simulink model "Ghost"  (Simulink 8.1)
settings: Solver=ode1  StartTime=0.0  StopTime=inf  FixedStep=Ts  MaxStep=1e-3  RelTol=1e-3
PostLoadFcn:
  | NREL_Mode=1; Ghost_init;
InitFcn:
  | NREL_Mode=1; Ghost_init;
undefined symbols (not defined in the file): Stim, Ts
libraries: simulink x75, artemis x11, relay_housing_lib x4, rtlab x1, utility_service_lib x1, communications_lib x1, Feeder1_lib x1, Feeder2_lib x1, Feeder3_lib x1, Feeder4_lib x1, powerlib x1
(part 2 of 2)

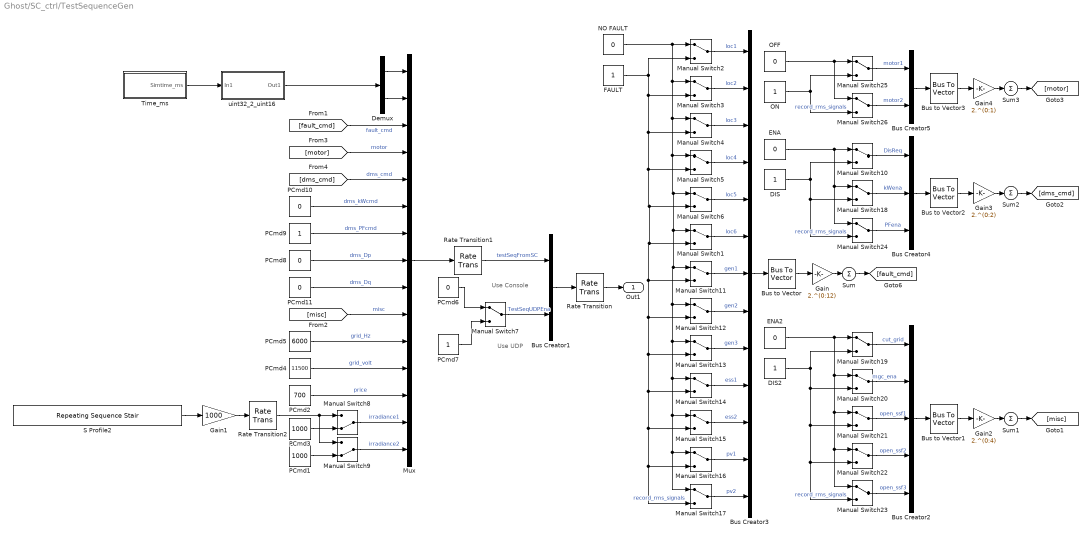
== system Ghost/SC_ctrl/TestSequenceGen ==
  note: Use UDP
  note: Use Console
  Bus Creator1 : BusCreator  Inputs=2
  Bus Creator2 : BusCreator  Inputs=5
  Bus Creator3 : BusCreator  Inputs=13
  Bus Creator4 : BusCreator  Inputs=3
  Bus Creator5 : BusCreator  Inputs=2
  Bus to Vector{,1..3} (4 alike) : BusToVector
  DIS : Constant
  DIS2 : Constant
  Demux : Demux  Outputs=2
  ENA : Constant  Value=0
  ENA2 : Constant  Value=0
  FAULT : Constant
  Gain : Gain  Gain=2.^(0:12)
  Gain1 : Gain  Gain=1000
  Gain2 : Gain  Gain=2.^(0:4)
  Gain3 : Gain  Gain=2.^(0:2)
  Gain4 : Gain  Gain=2.^(0:1)
  Manual Switch{1..7,10..26} (24 alike) : ManualSwitch
  Manual Switch8 : ManualSwitch  CurrentSetting=0
  Manual Switch9 : ManualSwitch  CurrentSetting=0
  Mux : Mux  Inputs=15
  NO FAULT : Constant  Value=0
  OFF : Constant  Value=0
  ON : Constant
  PCmd1 : Constant  Value=1000
  PCmd10 : Constant  Value=0
  PCmd11 : Constant  Value=0
  PCmd2 : Constant  Value=700
  PCmd3 : Constant  Value=1000
  PCmd4 : Constant  Value=11500
  PCmd5 : Constant  Value=6000
  PCmd6 : Constant  Value=0  SampleTime=[Stim.Ts Ts]
  PCmd7 : Constant
  PCmd8 : Constant  Value=0
  PCmd9 : Constant
  Rate Transition : RateTransition  Deterministic=off
  Rate Transition1 : RateTransition  Deterministic=off  OutPortSampleTime=10e-3
  Rate Transition2 : RateTransition  Deterministic=off  OutPortSampleTime=10e-3
  S Profile2 : simulink/Sources/Repeating Sequence Stair  OutValues=Stim.PV2.Irradiance  tsamp=[Stim.Ts Ts]  OutMin=[]  OutMax=[]  OutDataTypeStr=Inherit: Inherit via back propagation  OutDataType=fixdt(0,8)  ConRadixGroup=Best Precision: Vector-wise  OutScaling=2^-12
  Sum{,1..3} (4 alike) : Sum  Inputs=+
  Time_ms : Subsystem
  uint32_2_uint16 : Subsystem
      mask Display: disp('uint32_2_uint16');
  Out1 : Outport
  wires:
  Rate Transition1/1 -> Bus Creator1/1  "testSeqFromSC"
  uint32_2_uint16/1(Out1) -> Demux/1
  S Profile2/1 -> Gain1/1
  Sum3/1 -> [motor]
  Gain4/1 -> Sum3/1
  Bus to Vector3/1 -> Gain4/1
  OFF/1 -> Manual Switch26/1, Manual Switch25/1
  ON/1 -> Manual Switch25/2, Manual Switch26/2  "record_rms_signals"
  Manual Switch26/1 -> Bus Creator5/2  "motor2"
  Manual Switch25/1 -> Bus Creator5/1  "motor1"
  Bus Creator5/1 -> Bus to Vector3/1
  Sum2/1 -> [dms_cmd]
  Gain3/1 -> Sum2/1
  Bus to Vector2/1 -> Gain3/1
  ENA/1 -> Manual Switch10/1, Manual Switch18/1, Manual Switch24/1
  DIS/1 -> Manual Switch18/2, Manual Switch24/2, Manual Switch10/2  "record_rms_signals"
  Manual Switch18/1 -> Bus Creator4/2  "kWena"
  Manual Switch10/1 -> Bus Creator4/1  "DisReq"
  Bus Creator4/1 -> Bus to Vector2/1
  Manual Switch24/1 -> Bus Creator4/3  "PFena"
  Sum1/1 -> [misc]
  Gain2/1 -> Sum1/1
  Bus to Vector1/1 -> Gain2/1
  ENA2/1 -> Manual Switch23/1, Manual Switch22/1, Manual Switch21/1, Manual Switch20/1, Manual Switch19/1
  DIS2/1 -> Manual Switch19/2, Manual Switch23/2, Manual Switch22/2, Manual Switch21/2, Manual Switch20/2  "record_rms_signals"
  Manual Switch20/1 -> Bus Creator2/2  "mgc_ena"
  Manual Switch23/1 -> Bus Creator2/5  "open_ssf3"
  Manual Switch19/1 -> Bus Creator2/1  "cut_grid"
  Bus Creator2/1 -> Bus to Vector1/1
  Manual Switch22/1 -> Bus Creator2/4  "open_ssf2"
  Manual Switch21/1 -> Bus Creator2/3  "open_ssf1"
  PCmd11/1 -> Mux/9  "dms_Dq"
  PCmd10/1 -> Mux/6  "dms_kWcmd"
  PCmd9/1 -> Mux/7  "dms_PFcmd"
  PCmd8/1 -> Mux/8  "dms_Dp"
  [dms_cmd] -> Mux/5  "dms_cmd"
  [motor] -> Mux/4  "motor"
  [misc] -> Mux/10  "misc"
  PCmd5/1 -> Mux/11  "grid_Hz"
  PCmd4/1 -> Mux/12  "grid_volt"
  Demux/2 -> Mux/2
  Demux/1 -> Mux/1
  Time_ms/1(Simtime_ms) -> uint32_2_uint16/1(In1)
  Gain1/1 -> Rate Transition2/1
  PCmd2/1 -> Mux/13  "price"
  Manual Switch8/1 -> Mux/14  "irradiance1"
  PCmd1/1 -> Manual Switch9/2
  Manual Switch9/1 -> Mux/15  "irradiance2"
  PCmd3/1 -> Manual Switch8/2
  Rate Transition/1 -> Out1/1
  PCmd7/1 -> Manual Switch7/2
  PCmd6/1 -> Manual Switch7/1
  Manual Switch7/1 -> Bus Creator1/2  "TestSeqUDPEna"
  Bus Creator1/1 -> Rate Transition/1
  Mux/1 -> Rate Transition1/1
  Sum/1 -> [fault_cmd]
  Gain/1 -> Sum/1
  Bus to Vector/1 -> Gain/1
  Manual Switch17/1 -> Bus Creator3/13  "pv2"
  Manual Switch16/1 -> Bus Creator3/12  "pv1"
  NO FAULT/1 -> Manual Switch2/1, Manual Switch3/1, Manual Switch4/1, Manual Switch5/1, Manual Switch6/1, Manual Switch1/1, Manual Switch11/1, Manual Switch16/1, Manual Switch17/1, Manual Switch15/1, Manual Switch14/1, Manual Switch13/1, Manual Switch12/1
  FAULT/1 -> Manual Switch3/2, Manual Switch4/2, Manual Switch5/2, Manual Switch6/2, Manual Switch11/2, Manual Switch15/2, Manual Switch16/2, Manual Switch17/2, Manual Switch14/2, Manual Switch13/2, Manual Switch12/2, Manual Switch1/2, Manual Switch2/2  "record_rms_signals"
  Manual Switch12/1 -> Bus Creator3/8  "gen2"
  Manual Switch15/1 -> Bus Creator3/11  "ess2"
  Manual Switch11/1 -> Bus Creator3/7  "gen1"
  Manual Switch14/1 -> Bus Creator3/10  "ess1"
  Manual Switch13/1 -> Bus Creator3/9  "gen3"
  Manual Switch1/1 -> Bus Creator3/6  "loc6"
  Manual Switch3/1 -> Bus Creator3/2  "loc2"
  Manual Switch6/1 -> Bus Creator3/5  "loc5"
  Manual Switch2/1 -> Bus Creator3/1  "loc1"
  Bus Creator3/1 -> Bus to Vector/1
  [fault_cmd] -> Mux/3  "fault_cmd"
  Manual Switch5/1 -> Bus Creator3/4  "loc4"
  Manual Switch4/1 -> Bus Creator3/3  "loc3"
  Rate Transition2/1 -> Manual Switch8/1, Manual Switch9/1

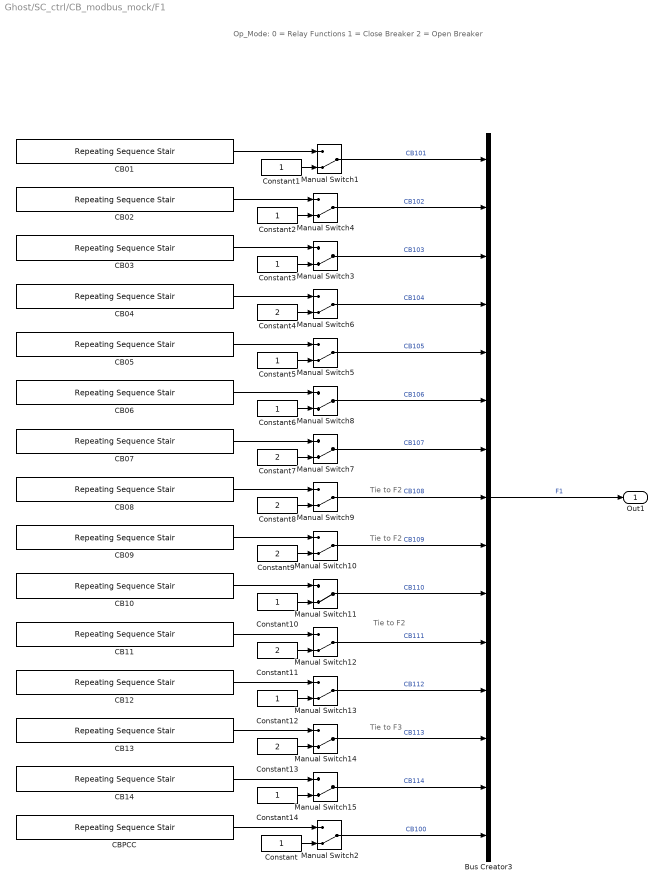
== system Ghost/SC_ctrl/CB_modbus_mock/F1 ==
  note: Tie to F2
  note: Tie to F2
  note: Op_Mode:
      | 0 = Relay Functions
      | 1 = Close Breaker
      | 2 = Open Breaker
  note: Tie to F2
  note: Tie to F3
  Bus Creator3 : BusCreator  Inputs=15
  CB01 : simulink/Sources/Repeating Sequence Stair  OutValues=Stim.CB.CB101  tsamp=[Stim.Ts Ts]  OutMin=[]  OutMax=[]  OutDataTypeStr=Inherit: Inherit via back propagation  OutDataType=fixdt(0,8)  ConRadixGroup=Best Precision: Vector-wise  OutScaling=2^-12
  CB02 : simulink/Sources/Repeating Sequence Stair  OutValues=Stim.CB.CB102  tsamp=[Stim.Ts Ts]  OutMin=[]  OutMax=[]  OutDataTypeStr=Inherit: Inherit via back propagation  OutDataType=fixdt(0,8)  ConRadixGroup=Best Precision: Vector-wise  OutScaling=2^-12
  CB03 : simulink/Sources/Repeating Sequence Stair  OutValues=Stim.CB.CB103  tsamp=[Stim.Ts Ts]  OutMin=[]  OutMax=[]  OutDataTypeStr=Inherit: Inherit via back propagation  OutDataType=fixdt(0,8)  ConRadixGroup=Best Precision: Vector-wise  OutScaling=2^-12
  CB04 : simulink/Sources/Repeating Sequence Stair  OutValues=Stim.CB.CB104  tsamp=[Stim.Ts Ts]  OutMin=[]  OutMax=[]  OutDataTypeStr=Inherit: Inherit via back propagation  OutDataType=fixdt(0,8)  ConRadixGroup=Best Precision: Vector-wise  OutScaling=2^-12
  CB05 : simulink/Sources/Repeating Sequence Stair  OutValues=Stim.CB.CB105  tsamp=[Stim.Ts Ts]  OutMin=[]  OutMax=[]  OutDataTypeStr=Inherit: Inherit via back propagation  OutDataType=fixdt(0,8)  ConRadixGroup=Best Precision: Vector-wise  OutScaling=2^-12
  CB06 : simulink/Sources/Repeating Sequence Stair  OutValues=Stim.CB.CB106  tsamp=[Stim.Ts Ts]  OutMin=[]  OutMax=[]  OutDataTypeStr=Inherit: Inherit via back propagation  OutDataType=fixdt(0,8)  ConRadixGroup=Best Precision: Vector-wise  OutScaling=2^-12
  CB07 : simulink/Sources/Repeating Sequence Stair  OutValues=Stim.CB.CB107  tsamp=[Stim.Ts Ts]  OutMin=[]  OutMax=[]  OutDataTypeStr=Inherit: Inherit via back propagation  OutDataType=fixdt(0,8)  ConRadixGroup=Best Precision: Vector-wise  OutScaling=2^-12
  CB08 : simulink/Sources/Repeating Sequence Stair  OutValues=Stim.CB.CB108  tsamp=[Stim.Ts Ts]  OutMin=[]  OutMax=[]  OutDataTypeStr=Inherit: Inherit via back propagation  OutDataType=fixdt(0,8)  ConRadixGroup=Best Precision: Vector-wise  OutScaling=2^-12
  CB09 : simulink/Sources/Repeating Sequence Stair  OutValues=Stim.CB.CB109  tsamp=[Stim.Ts Ts]  OutMin=[]  OutMax=[]  OutDataTypeStr=Inherit: Inherit via back propagation  OutDataType=fixdt(0,8)  ConRadixGroup=Best Precision: Vector-wise  OutScaling=2^-12
  CB10 : simulink/Sources/Repeating Sequence Stair  OutValues=Stim.CB.CB110  tsamp=[Stim.Ts Ts]  OutMin=[]  OutMax=[]  OutDataTypeStr=Inherit: Inherit via back propagation  OutDataType=fixdt(0,8)  ConRadixGroup=Best Precision: Vector-wise  OutScaling=2^-12
  CB11 : simulink/Sources/Repeating Sequence Stair  OutValues=Stim.CB.CB111  tsamp=[Stim.Ts Ts]  OutMin=[]  OutMax=[]  OutDataTypeStr=Inherit: Inherit via back propagation  OutDataType=fixdt(0,8)  ConRadixGroup=Best Precision: Vector-wise  OutScaling=2^-12
  CB12 : simulink/Sources/Repeating Sequence Stair  OutValues=Stim.CB.CB112  tsamp=[Stim.Ts Ts]  OutMin=[]  OutMax=[]  OutDataTypeStr=Inherit: Inherit via back propagation  OutDataType=fixdt(0,8)  ConRadixGroup=Best Precision: Vector-wise  OutScaling=2^-12
  CB13 : simulink/Sources/Repeating Sequence Stair  OutValues=Stim.CB.CB113  tsamp=[Stim.Ts Ts]  OutMin=[]  OutMax=[]  OutDataTypeStr=Inherit: Inherit via back propagation  OutDataType=fixdt(0,8)  ConRadixGroup=Best Precision: Vector-wise  OutScaling=2^-12
  CB14 : simulink/Sources/Repeating Sequence Stair  OutValues=Stim.CB.CB114  tsamp=[Stim.Ts Ts]  OutMin=[]  OutMax=[]  OutDataTypeStr=Inherit: Inherit via back propagation  OutDataType=fixdt(0,8)  ConRadixGroup=Best Precision: Vector-wise  OutScaling=2^-12
  CBPCC : simulink/Sources/Repeating Sequence Stair  OutValues=Stim.CB.CB100  tsamp=[Stim.Ts Ts]  OutMin=[]  OutMax=[]  OutDataTypeStr=Inherit: Inherit via back propagation  OutDataType=fixdt(0,8)  ConRadixGroup=Best Precision: Vector-wise  OutScaling=2^-12
  Constant{,1..3,5..6,10,12,14} (9 alike) : Constant
  Constant{4,7..9,11,13} (6 alike) : Constant  Value=2
  Manual Switch{1..15} (15 alike) : ManualSwitch  CurrentSetting=0
  Out1 : Outport
  wires:
  CB08/1 -> Manual Switch9/1
  Constant8/1 -> Manual Switch9/2
  Constant9/1 -> Manual Switch10/2
  Manual Switch9/1 -> Bus Creator3/8  "CB108"
  CB02/1 -> Manual Switch4/1
  Constant1/1 -> Manual Switch1/2
  Constant7/1 -> Manual Switch7/2
  Constant6/1 -> Manual Switch8/2
  CB07/1 -> Manual Switch7/1
  CB09/1 -> Manual Switch10/1
  Constant2/1 -> Manual Switch4/2
  CB06/1 -> Manual Switch8/1
  CB05/1 -> Manual Switch5/1
  Constant4/1 -> Manual Switch6/2
  Constant5/1 -> Manual Switch5/2
  CB04/1 -> Manual Switch6/1
  Manual Switch10/1 -> Bus Creator3/9  "CB109"
  Manual Switch8/1 -> Bus Creator3/6  "CB106"
  Manual Switch5/1 -> Bus Creator3/5  "CB105"
  Manual Switch6/1 -> Bus Creator3/4  "CB104"
  Manual Switch4/1 -> Bus Creator3/2  "CB102"
  Manual Switch1/1 -> Bus Creator3/1  "CB101"
  Manual Switch3/1 -> Bus Creator3/3  "CB103"
  Manual Switch7/1 -> Bus Creator3/7  "CB107"
  Manual Switch2/1 -> Bus Creator3/15  "CB100"
  Constant/1 -> Manual Switch2/2
  CBPCC/1 -> Manual Switch2/1
  CB01/1 -> Manual Switch1/1
  Bus Creator3/1 -> Out1/1  "F1"
  CB03/1 -> Manual Switch3/1
  Constant3/1 -> Manual Switch3/2
  Constant10/1 -> Manual Switch11/2
  CB10/1 -> Manual Switch11/1
  Manual Switch11/1 -> Bus Creator3/10  "CB110"
  Constant11/1 -> Manual Switch12/2
  CB11/1 -> Manual Switch12/1
  Manual Switch12/1 -> Bus Creator3/11  "CB111"
  Constant12/1 -> Manual Switch13/2
  CB12/1 -> Manual Switch13/1
  Manual Switch13/1 -> Bus Creator3/12  "CB112"
  Constant13/1 -> Manual Switch14/2
  CB13/1 -> Manual Switch14/1
  Manual Switch14/1 -> Bus Creator3/13  "CB113"
  Constant14/1 -> Manual Switch15/2
  CB14/1 -> Manual Switch15/1
  Manual Switch15/1 -> Bus Creator3/14  "CB114"

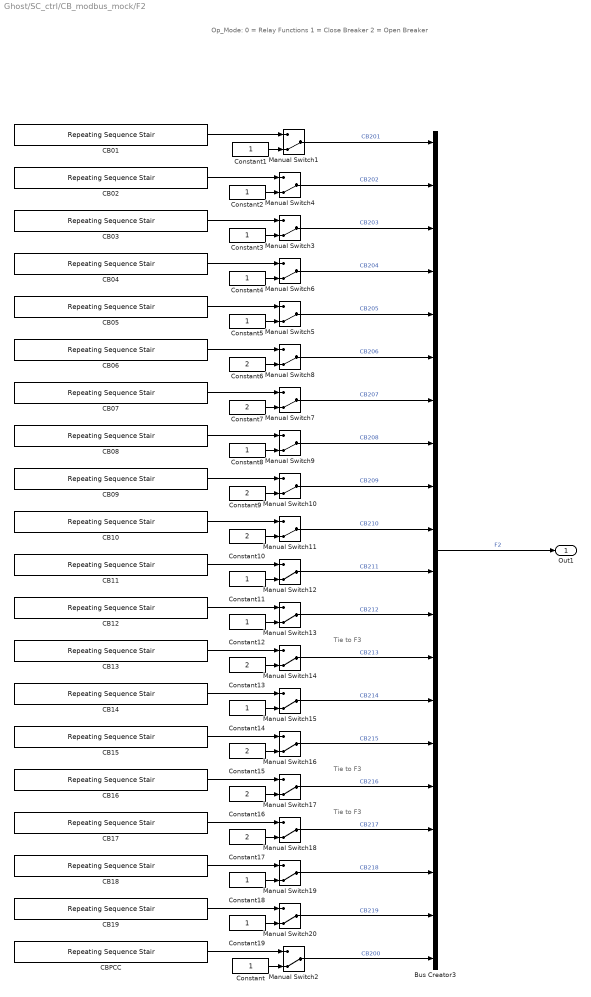
== system Ghost/SC_ctrl/CB_modbus_mock/F2 ==
  note: Tie to F3
  note: Op_Mode:
      | 0 = Relay Functions
      | 1 = Close Breaker
      | 2 = Open Breaker
  note: Tie to F3
  note: Tie to F3
  Bus Creator3 : BusCreator  Inputs=20
  CB01 : simulink/Sources/Repeating Sequence Stair  OutValues=Stim.CB.CB201  tsamp=[Stim.Ts Ts]  OutMin=[]  OutMax=[]  OutDataTypeStr=Inherit: Inherit via back propagation  OutDataType=fixdt(0,8)  ConRadixGroup=Best Precision: Vector-wise  OutScaling=2^-12
  CB02 : simulink/Sources/Repeating Sequence Stair  OutValues=Stim.CB.CB202  tsamp=[Stim.Ts Ts]  OutMin=[]  OutMax=[]  OutDataTypeStr=Inherit: Inherit via back propagation  OutDataType=fixdt(0,8)  ConRadixGroup=Best Precision: Vector-wise  OutScaling=2^-12
  CB03 : simulink/Sources/Repeating Sequence Stair  OutValues=Stim.CB.CB203  tsamp=[Stim.Ts Ts]  OutMin=[]  OutMax=[]  OutDataTypeStr=Inherit: Inherit via back propagation  OutDataType=fixdt(0,8)  ConRadixGroup=Best Precision: Vector-wise  OutScaling=2^-12
  CB04 : simulink/Sources/Repeating Sequence Stair  OutValues=Stim.CB.CB204  tsamp=[Stim.Ts Ts]  OutMin=[]  OutMax=[]  OutDataTypeStr=Inherit: Inherit via back propagation  OutDataType=fixdt(0,8)  ConRadixGroup=Best Precision: Vector-wise  OutScaling=2^-12
  CB05 : simulink/Sources/Repeating Sequence Stair  OutValues=Stim.CB.CB205  tsamp=[Stim.Ts Ts]  OutMin=[]  OutMax=[]  OutDataTypeStr=Inherit: Inherit via back propagation  OutDataType=fixdt(0,8)  ConRadixGroup=Best Precision: Vector-wise  OutScaling=2^-12
  CB06 : simulink/Sources/Repeating Sequence Stair  OutValues=Stim.CB.CB206  tsamp=[Stim.Ts Ts]  OutMin=[]  OutMax=[]  OutDataTypeStr=Inherit: Inherit via back propagation  OutDataType=fixdt(0,8)  ConRadixGroup=Best Precision: Vector-wise  OutScaling=2^-12
  CB07 : simulink/Sources/Repeating Sequence Stair  OutValues=Stim.CB.CB207  tsamp=[Stim.Ts Ts]  OutMin=[]  OutMax=[]  OutDataTypeStr=Inherit: Inherit via back propagation  OutDataType=fixdt(0,8)  ConRadixGroup=Best Precision: Vector-wise  OutScaling=2^-12
  CB08 : simulink/Sources/Repeating Sequence Stair  OutValues=Stim.CB.CB208  tsamp=[Stim.Ts Ts]  OutMin=[]  OutMax=[]  OutDataTypeStr=Inherit: Inherit via back propagation  OutDataType=fixdt(0,8)  ConRadixGroup=Best Precision: Vector-wise  OutScaling=2^-12
  CB09 : simulink/Sources/Repeating Sequence Stair  OutValues=Stim.CB.CB209  tsamp=[Stim.Ts Ts]  OutMin=[]  OutMax=[]  OutDataTypeStr=Inherit: Inherit via back propagation  OutDataType=fixdt(0,8)  ConRadixGroup=Best Precision: Vector-wise  OutScaling=2^-12
  CB10 : simulink/Sources/Repeating Sequence Stair  OutValues=Stim.CB.CB210  tsamp=[Stim.Ts Ts]  OutMin=[]  OutMax=[]  OutDataTypeStr=Inherit: Inherit via back propagation  OutDataType=fixdt(0,8)  ConRadixGroup=Best Precision: Vector-wise  OutScaling=2^-12
  CB11 : simulink/Sources/Repeating Sequence Stair  OutValues=Stim.CB.CB211  tsamp=[Stim.Ts Ts]  OutMin=[]  OutMax=[]  OutDataTypeStr=Inherit: Inherit via back propagation  OutDataType=fixdt(0,8)  ConRadixGroup=Best Precision: Vector-wise  OutScaling=2^-12
  CB12 : simulink/Sources/Repeating Sequence Stair  OutValues=Stim.CB.CB212  tsamp=[Stim.Ts Ts]  OutMin=[]  OutMax=[]  OutDataTypeStr=Inherit: Inherit via back propagation  OutDataType=fixdt(0,8)  ConRadixGroup=Best Precision: Vector-wise  OutScaling=2^-12
  CB13 : simulink/Sources/Repeating Sequence Stair  OutValues=Stim.CB.CB213  tsamp=[Stim.Ts Ts]  OutMin=[]  OutMax=[]  OutDataTypeStr=Inherit: Inherit via back propagation  OutDataType=fixdt(0,8)  ConRadixGroup=Best Precision: Vector-wise  OutScaling=2^-12
  CB14 : simulink/Sources/Repeating Sequence Stair  OutValues=Stim.CB.CB214  tsamp=[Stim.Ts Ts]  OutMin=[]  OutMax=[]  OutDataTypeStr=Inherit: Inherit via back propagation  OutDataType=fixdt(0,8)  ConRadixGroup=Best Precision: Vector-wise  OutScaling=2^-12
  CB15 : simulink/Sources/Repeating Sequence Stair  OutValues=Stim.CB.CB215  tsamp=[Stim.Ts Ts]  OutMin=[]  OutMax=[]  OutDataTypeStr=Inherit: Inherit via back propagation  OutDataType=fixdt(0,8)  ConRadixGroup=Best Precision: Vector-wise  OutScaling=2^-12
  CB16 : simulink/Sources/Repeating Sequence Stair  OutValues=Stim.CB.CB216  tsamp=[Stim.Ts Ts]  OutMin=[]  OutMax=[]  OutDataTypeStr=Inherit: Inherit via back propagation  OutDataType=fixdt(0,8)  ConRadixGroup=Best Precision: Vector-wise  OutScaling=2^-12
  CB17 : simulink/Sources/Repeating Sequence Stair  OutValues=Stim.CB.CB217  tsamp=[Stim.Ts Ts]  OutMin=[]  OutMax=[]  OutDataTypeStr=Inherit: Inherit via back propagation  OutDataType=fixdt(0,8)  ConRadixGroup=Best Precision: Vector-wise  OutScaling=2^-12
  CB18 : simulink/Sources/Repeating Sequence Stair  OutValues=Stim.CB.CB218  tsamp=[Stim.Ts Ts]  OutMin=[]  OutMax=[]  OutDataTypeStr=Inherit: Inherit via back propagation  OutDataType=fixdt(0,8)  ConRadixGroup=Best Precision: Vector-wise  OutScaling=2^-12
  CB19 : simulink/Sources/Repeating Sequence Stair  OutValues=Stim.CB.CB219  tsamp=[Stim.Ts Ts]  OutMin=[]  OutMax=[]  OutDataTypeStr=Inherit: Inherit via back propagation  OutDataType=fixdt(0,8)  ConRadixGroup=Best Precision: Vector-wise  OutScaling=2^-12
  CBPCC : simulink/Sources/Repeating Sequence Stair  OutValues=Stim.CB.CB200  tsamp=[Stim.Ts Ts]  OutMin=[]  OutMax=[]  OutDataTypeStr=Inherit: Inherit via back propagation  OutDataType=fixdt(0,8)  ConRadixGroup=Best Precision: Vector-wise  OutScaling=2^-12
  Constant{,1..5,8,11..12,14,18..19} (12 alike) : Constant
  Constant{6..7,9..10,13,15..17} (8 alike) : Constant  Value=2
  Manual Switch{1..20} (20 alike) : ManualSwitch  CurrentSetting=0
  Out1 : Outport
  wires:
  Manual Switch15/1 -> Bus Creator3/14  "CB214"
  CB14/1 -> Manual Switch15/1
  Constant14/1 -> Manual Switch15/2
  Manual Switch14/1 -> Bus Creator3/13  "CB213"
  CB13/1 -> Manual Switch14/1
  Constant13/1 -> Manual Switch14/2
  Manual Switch13/1 -> Bus Creator3/12  "CB212"
  CB12/1 -> Manual Switch13/1
  Constant12/1 -> Manual Switch13/2
  Manual Switch12/1 -> Bus Creator3/11  "CB211"
  CB11/1 -> Manual Switch12/1
  Constant11/1 -> Manual Switch12/2
  Manual Switch11/1 -> Bus Creator3/10  "CB210"
  CB10/1 -> Manual Switch11/1
  Constant10/1 -> Manual Switch11/2
  Constant3/1 -> Manual Switch3/2
  CB03/1 -> Manual Switch3/1
  Bus Creator3/1 -> Out1/1  "F2"
  CB01/1 -> Manual Switch1/1
  CBPCC/1 -> Manual Switch2/1
  Constant/1 -> Manual Switch2/2
  Manual Switch2/1 -> Bus Creator3/20  "CB200"
  Manual Switch7/1 -> Bus Creator3/7  "CB207"
  Manual Switch3/1 -> Bus Creator3/3  "CB203"
  Manual Switch1/1 -> Bus Creator3/1  "CB201"
  Manual Switch4/1 -> Bus Creator3/2  "CB202"
  Manual Switch6/1 -> Bus Creator3/4  "CB204"
  Manual Switch5/1 -> Bus Creator3/5  "CB205"
  Manual Switch8/1 -> Bus Creator3/6  "CB206"
  Manual Switch10/1 -> Bus Creator3/9  "CB209"
  CB04/1 -> Manual Switch6/1
  Constant5/1 -> Manual Switch5/2
  Constant4/1 -> Manual Switch6/2
  CB05/1 -> Manual Switch5/1
  CB06/1 -> Manual Switch8/1
  Constant2/1 -> Manual Switch4/2
  CB09/1 -> Manual Switch10/1
  CB07/1 -> Manual Switch7/1
  Constant6/1 -> Manual Switch8/2
  Constant7/1 -> Manual Switch7/2
  Constant1/1 -> Manual Switch1/2
  CB02/1 -> Manual Switch4/1
  Manual Switch9/1 -> Bus Creator3/8  "CB208"
  Constant9/1 -> Manual Switch10/2
  Constant8/1 -> Manual Switch9/2
  CB08/1 -> Manual Switch9/1
  Manual Switch20/1 -> Bus Creator3/19  "CB219"
  CB19/1 -> Manual Switch20/1
  Constant19/1 -> Manual Switch20/2
  Manual Switch19/1 -> Bus Creator3/18  "CB218"
  CB18/1 -> Manual Switch19/1
  Constant18/1 -> Manual Switch19/2
  Manual Switch18/1 -> Bus Creator3/17  "CB217"
  CB17/1 -> Manual Switch18/1
  Constant17/1 -> Manual Switch18/2
  Manual Switch17/1 -> Bus Creator3/16  "CB216"
  CB16/1 -> Manual Switch17/1
  Constant16/1 -> Manual Switch17/2
  Manual Switch16/1 -> Bus Creator3/15  "CB215"
  CB15/1 -> Manual Switch16/1
  Constant15/1 -> Manual Switch16/2

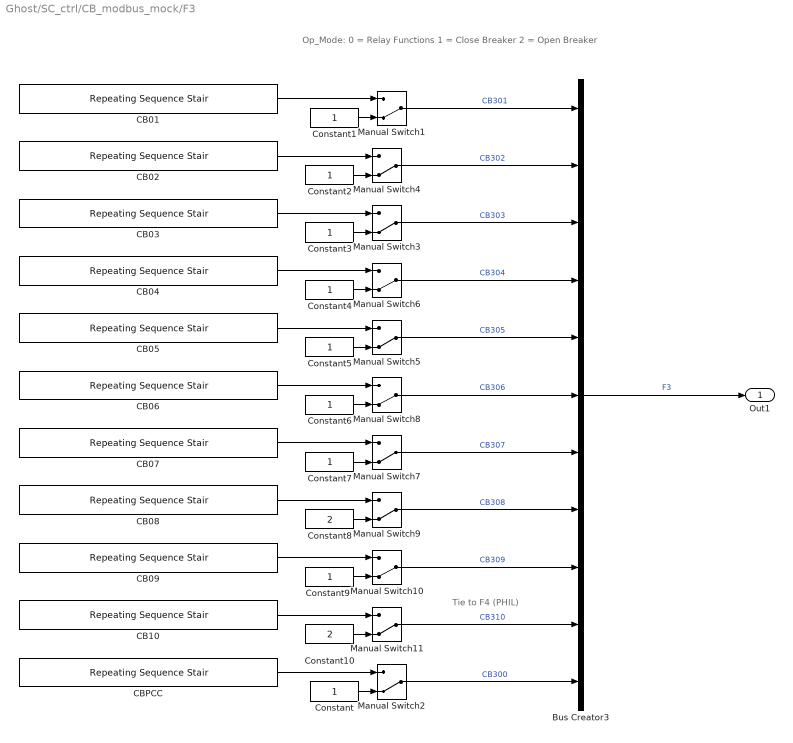
== system Ghost/SC_ctrl/CB_modbus_mock/F3 ==
  note: Tie to F4 (PHIL)
  note: Op_Mode:
      | 0 = Relay Functions
      | 1 = Close Breaker
      | 2 = Open Breaker
  Bus Creator3 : BusCreator  Inputs=11
  CB01 : simulink/Sources/Repeating Sequence Stair  OutValues=Stim.CB.CB301  tsamp=[Stim.Ts Ts]  OutMin=[]  OutMax=[]  OutDataTypeStr=Inherit: Inherit via back propagation  OutDataType=fixdt(0,8)  ConRadixGroup=Best Precision: Vector-wise  OutScaling=2^-12
  CB02 : simulink/Sources/Repeating Sequence Stair  OutValues=Stim.CB.CB302  tsamp=[Stim.Ts Ts]  OutMin=[]  OutMax=[]  OutDataTypeStr=Inherit: Inherit via back propagation  OutDataType=fixdt(0,8)  ConRadixGroup=Best Precision: Vector-wise  OutScaling=2^-12
  CB03 : simulink/Sources/Repeating Sequence Stair  OutValues=Stim.CB.CB303  tsamp=[Stim.Ts Ts]  OutMin=[]  OutMax=[]  OutDataTypeStr=Inherit: Inherit via back propagation  OutDataType=fixdt(0,8)  ConRadixGroup=Best Precision: Vector-wise  OutScaling=2^-12
  CB04 : simulink/Sources/Repeating Sequence Stair  OutValues=Stim.CB.CB304  tsamp=[Stim.Ts Ts]  OutMin=[]  OutMax=[]  OutDataTypeStr=Inherit: Inherit via back propagation  OutDataType=fixdt(0,8)  ConRadixGroup=Best Precision: Vector-wise  OutScaling=2^-12
  CB05 : simulink/Sources/Repeating Sequence Stair  OutValues=Stim.CB.CB305  tsamp=[Stim.Ts Ts]  OutMin=[]  OutMax=[]  OutDataTypeStr=Inherit: Inherit via back propagation  OutDataType=fixdt(0,8)  ConRadixGroup=Best Precision: Vector-wise  OutScaling=2^-12
  CB06 : simulink/Sources/Repeating Sequence Stair  OutValues=Stim.CB.CB306  tsamp=[Stim.Ts Ts]  OutMin=[]  OutMax=[]  OutDataTypeStr=Inherit: Inherit via back propagation  OutDataType=fixdt(0,8)  ConRadixGroup=Best Precision: Vector-wise  OutScaling=2^-12
  CB07 : simulink/Sources/Repeating Sequence Stair  OutValues=Stim.CB.CB307  tsamp=[Stim.Ts Ts]  OutMin=[]  OutMax=[]  OutDataTypeStr=Inherit: Inherit via back propagation  OutDataType=fixdt(0,8)  ConRadixGroup=Best Precision: Vector-wise  OutScaling=2^-12
  CB08 : simulink/Sources/Repeating Sequence Stair  OutValues=Stim.CB.CB308  tsamp=[Stim.Ts Ts]  OutMin=[]  OutMax=[]  OutDataTypeStr=Inherit: Inherit via back propagation  OutDataType=fixdt(0,8)  ConRadixGroup=Best Precision: Vector-wise  OutScaling=2^-12
  CB09 : simulink/Sources/Repeating Sequence Stair  OutValues=Stim.CB.CB309  tsamp=[Stim.Ts Ts]  OutMin=[]  OutMax=[]  OutDataTypeStr=Inherit: Inherit via back propagation  OutDataType=fixdt(0,8)  ConRadixGroup=Best Precision: Vector-wise  OutScaling=2^-12
  CB10 : simulink/Sources/Repeating Sequence Stair  OutValues=Stim.CB.CB310  tsamp=[Stim.Ts Ts]  OutMin=[]  OutMax=[]  OutDataTypeStr=Inherit: Inherit via back propagation  OutDataType=fixdt(0,8)  ConRadixGroup=Best Precision: Vector-wise  OutScaling=2^-12
  CBPCC : simulink/Sources/Repeating Sequence Stair  OutValues=Stim.CB.CB300  tsamp=[Stim.Ts Ts]  OutMin=[]  OutMax=[]  OutDataTypeStr=Inherit: Inherit via back propagation  OutDataType=fixdt(0,8)  ConRadixGroup=Best Precision: Vector-wise  OutScaling=2^-12
  Constant{,1..7,9} (9 alike) : Constant
  Constant10 : Constant  Value=2
  Constant8 : Constant  Value=2
  Manual Switch{1..11} (11 alike) : ManualSwitch  CurrentSetting=0
  Out1 : Outport
  wires:
  CB08/1 -> Manual Switch9/1
  Constant8/1 -> Manual Switch9/2
  Constant9/1 -> Manual Switch10/2
  Manual Switch9/1 -> Bus Creator3/8  "CB308"
  CB02/1 -> Manual Switch4/1
  Constant1/1 -> Manual Switch1/2
  Constant7/1 -> Manual Switch7/2
  Constant6/1 -> Manual Switch8/2
  CB07/1 -> Manual Switch7/1
  CB09/1 -> Manual Switch10/1
  Constant2/1 -> Manual Switch4/2
  CB06/1 -> Manual Switch8/1
  CB05/1 -> Manual Switch5/1
  Constant4/1 -> Manual Switch6/2
  Constant5/1 -> Manual Switch5/2
  CB04/1 -> Manual Switch6/1
  Manual Switch10/1 -> Bus Creator3/9  "CB309"
  Manual Switch8/1 -> Bus Creator3/6  "CB306"
  Manual Switch5/1 -> Bus Creator3/5  "CB305"
  Manual Switch6/1 -> Bus Creator3/4  "CB304"
  Manual Switch4/1 -> Bus Creator3/2  "CB302"
  Manual Switch1/1 -> Bus Creator3/1  "CB301"
  Manual Switch3/1 -> Bus Creator3/3  "CB303"
  Manual Switch7/1 -> Bus Creator3/7  "CB307"
  Manual Switch2/1 -> Bus Creator3/11  "CB300"
  Constant/1 -> Manual Switch2/2
  CBPCC/1 -> Manual Switch2/1
  CB01/1 -> Manual Switch1/1
  Bus Creator3/1 -> Out1/1  "F3"
  CB03/1 -> Manual Switch3/1
  Constant3/1 -> Manual Switch3/2
  Constant10/1 -> Manual Switch11/2
  CB10/1 -> Manual Switch11/1
  Manual Switch11/1 -> Bus Creator3/10  "CB310"

== system Ghost/SC_ctrl/CB_modbus_mock/F4 ==
  note: Copyright © 2017 the Alliance for Sustainable Energy, LLC
      |
      | The above copyright notice and this permission notice shall be included in all copies or substantial portions of the Software.
      |
      | THE SOFTWARE IS PROVIDED "AS IS", WITHOUT WARRANTY OF ANY KIND, EXPRESS OR IMPLIED, INCLUDING
      | BUT NOT LIMITED TO THE WARRANTIES OF MERCHANTABILITY, FITNESS FOR A PARTICULAR PURPOSE AND
      | NONINFRINGEMENT. IN NO EVENT SHALL THE AUTHORS OR COPYRIGHT HOLDERS BE LIABLE FOR ANY CLAIM,
      |  DAMAGES OR OTHER LIABILITY, WHETHER IN AN ACTION OF CONTRACT, TORT OR OTHERWISE, ARISING FROM,
      | OUT OF OR IN CONNECTION WITH THE SOFTWARE OR THE USE OR OTHER DEALINGS IN THE SOFTWARE
  note: Op_Mode:
      | 0 = Relay Functions
      | 1 = Close Breaker
      | 2 = Open Breaker
  Bus Creator3 : BusCreator  Inputs=6
  CB401 : simulink/Sources/Repeating Sequence Stair  OutValues=Stim.CB.CB401  tsamp=[Stim.Ts Ts]  OutMin=[]  OutMax=[]  OutDataTypeStr=Inherit: Inherit via back propagation  OutDataType=fixdt(0,8)  ConRadixGroup=Best Precision: Vector-wise  OutScaling=2^-12
  CB402 : simulink/Sources/Repeating Sequence Stair  OutValues=Stim.CB.CB402  tsamp=[Stim.Ts Ts]  OutMin=[]  OutMax=[]  OutDataTypeStr=Inherit: Inherit via back propagation  OutDataType=fixdt(0,8)  ConRadixGroup=Best Precision: Vector-wise  OutScaling=2^-12
  CB403 : simulink/Sources/Repeating Sequence Stair  OutValues=Stim.CB.CB403  tsamp=[Stim.Ts Ts]  OutMin=[]  OutMax=[]  OutDataTypeStr=Inherit: Inherit via back propagation  OutDataType=fixdt(0,8)  ConRadixGroup=Best Precision: Vector-wise  OutScaling=2^-12
  CB404 : simulink/Sources/Repeating Sequence Stair  OutValues=Stim.CB.CB404  tsamp=[Stim.Ts Ts]  OutMin=[]  OutMax=[]  OutDataTypeStr=Inherit: Inherit via back propagation  OutDataType=fixdt(0,8)  ConRadixGroup=Best Precision: Vector-wise  OutScaling=2^-12
  CB405 : simulink/Sources/Repeating Sequence Stair  OutValues=Stim.CB.CB405  tsamp=[Stim.Ts Ts]  OutMin=[]  OutMax=[]  OutDataTypeStr=Inherit: Inherit via back propagation  OutDataType=fixdt(0,8)  ConRadixGroup=Best Precision: Vector-wise  OutScaling=2^-12
  CB406 : simulink/Sources/Repeating Sequence Stair  OutValues=Stim.CB.CB406  tsamp=[Stim.Ts Ts]  OutMin=[]  OutMax=[]  OutDataTypeStr=Inherit: Inherit via back propagation  OutDataType=fixdt(0,8)  ConRadixGroup=Best Precision: Vector-wise  OutScaling=2^-12
  Constant : Constant  Value=2
  Constant{1..5} (5 alike) : Constant  Value=0
  Manual Switch{1,3..6} (5 alike) : ManualSwitch
  Manual Switch2 : ManualSwitch  CurrentSetting=0
  Out1 : Outport
  wires:
  Constant5/1 -> Manual Switch6/2
  CB406/1 -> Manual Switch6/1
  Constant4/1 -> Manual Switch5/2
  CB405/1 -> Manual Switch5/1
  Constant3/1 -> Manual Switch4/2
  CB404/1 -> Manual Switch4/1
  Constant2/1 -> Manual Switch3/2
  CB403/1 -> Manual Switch3/1
  Constant1/1 -> Manual Switch1/2
  Manual Switch4/1 -> Bus Creator3/4  "CB404"
  Manual Switch3/1 -> Bus Creator3/3  "CB403"
  Manual Switch5/1 -> Bus Creator3/5  "CB405"
  Manual Switch1/1 -> Bus Creator3/2  "CB402"
  CB402/1 -> Manual Switch1/1
  Manual Switch6/1 -> Bus Creator3/6  "CB406"
  Manual Switch2/1 -> Bus Creator3/1  "CB401"
  Constant/1 -> Manual Switch2/2
  CB401/1 -> Manual Switch2/1
  Bus Creator3/1 -> Out1/1  "F4"

== system Ghost/SC_ctrl/PV1 control/Tuning ==
  note: Not applicable
      | for PV
  Bus Creator : BusCreator  Inputs=7
  Constant : Constant  Value=2  SampleTime=[Stim.Ts Ts]
  Constant1 : Constant  Value=0.6e-3  SampleTime=[Stim.Ts Ts]
  Constant2 : Constant  Value=180  SampleTime=[Stim.Ts Ts]
  Constant3 : Constant  Value=3200  SampleTime=[Stim.Ts Ts]
  Constant4 : Constant  SampleTime=[Stim.Ts Ts]
  Constant5 : Constant  SampleTime=[Stim.Ts Ts]
  Constant6 : Constant  SampleTime=[Stim.Ts Ts]
  Tuning : Outport
  wires:
  Constant4/1 -> Bus Creator/5  "vff_ena"
  Constant3/1 -> Bus Creator/4  "pll_ki"
  Constant2/1 -> Bus Creator/3  "pll_kp"
  Constant1/1 -> Bus Creator/2  "csi_Ti"
  Constant/1 -> Bus Creator/1  "csi_kp"
  Bus Creator/1 -> Tuning/1
  Constant5/1 -> Bus Creator/6  "batt_cap_div"
  Constant6/1 -> Bus Creator/7  "batt_soc_rst"

== system Ghost/SC_ctrl/PV2 control/Tuning ==
  note: Nominal Insulation = 1000W/m^2
  note: A
      | --------
      | W/m^2
  note: Not applicable
      | for PV
  Bus Creator : BusCreator  Inputs=13
  Constant : Constant  Value=2  SampleTime=[Stim.Ts Ts]
  Constant1 : Constant  Value=0.6e-3  SampleTime=[Stim.Ts Ts]
  Constant10 : Constant  Value=570
  Constant11 : Constant  Value=0.2
  Constant12 : Constant  Value=0
  Constant2 : Constant  Value=180  SampleTime=[Stim.Ts Ts]
  Constant3 : Constant  Value=3200  SampleTime=[Stim.Ts Ts]
  Constant4 : Constant  SampleTime=[Stim.Ts Ts]
  Constant5 : Constant  SampleTime=[Stim.Ts Ts]
  Constant6 : Constant  SampleTime=[Stim.Ts Ts]
  Constant7 : Constant  Value=29
  Constant8 : Constant  Value=37
  Constant9 : Constant  Value=2
  Tuning : Outport
  wires:
  Constant4/1 -> Bus Creator/5  "vff_ena"
  Constant3/1 -> Bus Creator/4  "pll_ki"
  Constant2/1 -> Bus Creator/3  "pll_kp"
  Constant1/1 -> Bus Creator/2  "csi_Ti"
  Constant/1 -> Bus Creator/1  "csi_kp"
  Bus Creator/1 -> Tuning/1
  Constant5/1 -> Bus Creator/6  "batt_cap_div"
  Constant6/1 -> Bus Creator/7  "batt_soc_rst"
  Constant8/1 -> Bus Creator/9  "ParallelN"
  Constant7/1 -> Bus Creator/8  "SeriesN"
  Constant9/1 -> Bus Creator/10  "Imin"
  Constant10/1 -> Bus Creator/11  "Vref"
  Constant12/1 -> Bus Creator/12  "ConstCurEna"
  Constant11/1 -> Bus Creator/13  "ConstCurGain"

== system Ghost/SC_ctrl/Plots/Subsystem ==
  In1 : Inport
  Data Type Conversion3 : DataTypeConversion  OutDataTypeStr=double
  Data Type Conversion6 : DataTypeConversion  OutDataTypeStr=uint16
  Extract Bits1 : simulink/Logic and Bit Operations/Extract Bits  bitsToExtract=Range of bits  numBits=8  bitIdxRange=1  outScalingMode=Treat bit field as an integer
  Out1 : Outport
  wires:
  Data Type Conversion6/1 -> Extract Bits1/1
  In1/1 -> Data Type Conversion6/1
  Data Type Conversion3/1 -> Out1/1
  Extract Bits1/1 -> Data Type Conversion3/1

== system Ghost/SC_ctrl/SOC1 control/Tuning ==
  Bus Creator : BusCreator  Inputs=7
  Constant : Constant  Value=2  SampleTime=[Stim.Ts Ts]
  Constant1 : Constant  Value=0.6e-3  SampleTime=[Stim.Ts Ts]
  Constant2 : Constant  Value=180  SampleTime=[Stim.Ts Ts]
  Constant3 : Constant  Value=3200  SampleTime=[Stim.Ts Ts]
  Constant4 : Constant  SampleTime=[Stim.Ts Ts]
  Constant5 : Constant  SampleTime=[Stim.Ts Ts]
  Constant6 : Constant  Value=0  SampleTime=[Stim.Ts Ts]
  Tuning : Outport
  wires:
  Constant4/1 -> Bus Creator/5  "vff_ena"
  Constant3/1 -> Bus Creator/4  "pll_ki"
  Constant2/1 -> Bus Creator/3  "pll_kp"
  Constant1/1 -> Bus Creator/2  "csi_Ti"
  Constant/1 -> Bus Creator/1  "csi_kp"
  Bus Creator/1 -> Tuning/1
  Constant5/1 -> Bus Creator/6  "batt_cap_div"
  Constant6/1 -> Bus Creator/7  "batt_soc_rst"

== system Ghost/SC_ctrl/SOC2 control/Tuning ==
  Bus Creator : BusCreator  Inputs=7
  Constant : Constant  Value=2  SampleTime=[Stim.Ts Ts]
  Constant1 : Constant  Value=0.6e-3  SampleTime=[Stim.Ts Ts]
  Constant2 : Constant  Value=180  SampleTime=[Stim.Ts Ts]
  Constant3 : Constant  Value=3200  SampleTime=[Stim.Ts Ts]
  Constant4 : Constant  SampleTime=[Stim.Ts Ts]
  Constant5 : Constant  SampleTime=[Stim.Ts Ts]
  Constant6 : Constant  Value=0  SampleTime=[Stim.Ts Ts]
  Tuning : Outport
  wires:
  Constant4/1 -> Bus Creator/5  "vff_ena"
  Constant3/1 -> Bus Creator/4  "pll_ki"
  Constant2/1 -> Bus Creator/3  "pll_kp"
  Constant1/1 -> Bus Creator/2  "csi_Ti"
  Constant/1 -> Bus Creator/1  "csi_kp"
  Bus Creator/1 -> Tuning/1
  Constant5/1 -> Bus Creator/6  "batt_cap_div"
  Constant6/1 -> Bus Creator/7  "batt_soc_rst"

== system Ghost/SC_ctrl/TestSequenceGen/Time_ms ==
  Constant4 : Constant  Value=10
  Sum : Sum  Inputs=++|
  Unit Delay : UnitDelay  SampleTime=10e-3
  Simtime_ms : Outport
  wires:
  Sum/1 -> Simtime_ms/1, Unit Delay/1
  Constant4/1 -> Sum/2
  Unit Delay/1 -> Sum/1

== system Ghost/SC_ctrl/TestSequenceGen/uint32_2_uint16 ==
  In1 : Inport
  Data Type Conversion : DataTypeConversion  OutDataTypeStr=uint32
  Data Type Conversion1 : DataTypeConversion  OutDataTypeStr=double
  Data Type Conversion2 : DataTypeConversion  OutDataTypeStr=double
  Extract Bits : simulink/Logic and Bit Operations/Extract Bits  bitsToExtract=Upper half  numBits=8  bitIdxRange=[0 7]  outScalingMode=Treat bit field as an integer
  Extract Bits1 : simulink/Logic and Bit Operations/Extract Bits  bitsToExtract=Lower half  numBits=8  bitIdxRange=[0 7]  outScalingMode=Preserve fixed-point scaling
  Mux : Mux  Inputs=2
  Out1 : Outport
  wires:
  Mux/1 -> Out1/1
  Extract Bits/1 -> Data Type Conversion1/1
  In1/1 -> Data Type Conversion/1
  Data Type Conversion/1 -> Extract Bits1/1, Extract Bits/1
  Data Type Conversion2/1 -> Mux/1
  Data Type Conversion1/1 -> Mux/2
  Extract Bits1/1 -> Data Type Conversion2/1
